simulink library "carnotUIBK"  (R2024b)
settings: Solver=VariableStepAuto  StartTime=0.0  StopTime=10.0  RelTol=1e-3  EnableMultiTasking=on
values from neighbouring files (symbols this model uses):
  area = area + room(kk).area    [THERMALZONE.m]
  boundary = BOUNDARY()    [BUILDING.m]
  building = obj    [BUILDING.m]
  C = zeros(1,length(d)+1)    [CONSTRUCTION.m]
  cp = str2num(value)    [CONSTRUCTION.m]
  pos = find(d_layer>0)    [CONSTRUCTION.m]
  rho = str2num(value)    [CONSTRUCTION.m]
  type = 1    [CONSTRUCTION.m]
  zone = obj.zone(ind)    [THERMALZONE.m]
undefined symbols (not defined in the file or in its folder): A, amb_factor, B, const, control, Dd, get_building, height, p, Qdot_C, Qdot_H, Qdot_I_electricity, Qdot_I_light, Qdot_I_person, Qdot_S, Qdot_T_ground, Qdot_T_neighbour, Qdot_T_opaque, Qdot_T_window, Qdot_V_infiltration, Qdot_V_mech, Qdot_V_window, r_frame, solar_ratio, solar_ratio1, solar_ratio2, Tc, Tr, Ts, Uvalue, view_factor, wall, wallsurface, window, window_height, window_heigth, window_width, windowsurface, x_CO2, x_H2O, x_VOC, z
libraries: carnot x105, $bdroot x22, simulink x18, simulink_extras x14
(part 13 of 13)

== system carnotUIBK/wall_zone/hygrothermal model/alpha_e/alpha_e_INTERNAL/alpha_i/alpha_i_down ==
  note: (W/m^2)
  note: Convective and radiative heat transfer at the INDOOR SURFACE of a VERTICAL OUTER WALL
  note: CONVENTION:
      | Qdot > 0 and qdots < 0, if Ts > T (heat flows from wall surface to room node),
      | Qdot < 0 and qdots > 0, if Ts < T (heat flows from room node to wall surface).
  note: s: surface
      | c: convective
      | r: radiative
  note: dynamic, convective heat transfer coefficients according to: Glück B.: Wärmeübergangskoeffizienten an thermisch aktiven Bauteiloberflächen
      | und der Übergang zu Basiskennlinien für die Wärmestromdichte; gi Gesundheits-Ingenieur; 128. Jahrgang 2007, Heft 1, Seiten 1-10
  Ts : Inport
  AIB : Inport  Port=2
  Qdot sol : Inport  Port=3
  phis : Inport  Port=4
  1/wallsurface : Gain  Gain=1/wallsurface  SaturateOnIntegerOverflow=on  OutDataTypeStr=Inherit: Same as input  ParamDataTypeStr=Inherit: Same as input
  Add : Sum  Commented=on  Inputs=+-
  Bus Selector : BusSelector  OutputSignals=Tc,Tr,p,x_H2O
  Fcn1 : Fcn  Expr=(273.15+u(1))^4-(273.15+u(2))^4
  Gain2 : Gain  Commented=on  Gain=0.01
  Ground1 : Ground
  Ground2 : Ground
  Ground3 : Ground
  Mux : Mux  Inputs=2
  Mux1 : Mux  Inputs=[2 2 1 2 12]
  Mux2 : Mux  Inputs=2
  Mux3 : Mux  Inputs=2
  Product : Product  InputSameDT=on  RndMeth=Zero  SaturateOnIntegerOverflow=on  OutDataTypeStr=Inherit: Same as first input
  Product1 : Product  InputSameDT=on  RndMeth=Zero  SaturateOnIntegerOverflow=on  OutDataTypeStr=Inherit: Same as first input
  Product2 : Product  Commented=on  RndMeth=Zero
  Product3 : Product  Commented=on  RndMeth=Zero
  Sum : Sum  Inputs=+-  InputSameDT=on  SaturateOnIntegerOverflow=on  OutDataTypeStr=Inherit: Same as first input
  Sum2 : Sum  Inputs=+--  InputSameDT=on  SaturateOnIntegerOverflow=on  OutDataTypeStr=Inherit: Same as first input
  Switch : Switch  Commented=on  Criteria=u2 > Threshold  SaturateOnIntegerOverflow=off  InputSameDT=off
  Switch1 : Switch  SaturateOnIntegerOverflow=off  InputSameDT=off
  emission_in : Gain  Gain=emission_in  SaturateOnIntegerOverflow=on  OutDataTypeStr=Inherit: Same as input  ParamDataTypeStr=Inherit: Same as input
  heat flux downwards : Fcn  Expr=0.54*(abs(u(1)-u(2))^0.31)
  heat flux upwards : Fcn  Expr=2*(abs(u(1)-u(2))^0.31)
  lewis : Gain  Commented=on  Gain=0.000000007  SaturateOnIntegerOverflow=on  OutDataTypeStr=Inherit: Same as input  ParamDataTypeStr=Inherit: Same as input
  nomassflow : Constant  Value=0
  ps_l : Fcn  Commented=on  Expr=610.0*exp(17.08*(u)/(234.2+(u)))
  ps_s_l : Fcn  Commented=on  Expr=610.0*exp(17.08*(u)/(234.2+(u)))
  sigma : Constant  Value=5.67e-8
  view_factor : Gain  Gain=view_factor  SaturateOnIntegerOverflow=on  OutDataTypeStr=Inherit: Same as input  ParamDataTypeStr=Inherit: Same as input
  wallsurface : Gain  Gain=wallsurface  SaturateOnIntegerOverflow=on  OutDataTypeStr=Inherit: Same as input  ParamDataTypeStr=Inherit: Same as input
  wallsurface1 : Gain  Commented=on  Gain=wallsurface  SaturateOnIntegerOverflow=on  OutDataTypeStr=Inherit: Same as input  ParamDataTypeStr=Inherit: Same as input
  x2RelHum_UIBK : carnot/Basic/Material_Properties/x2RelHum  Commented=on
      settings: SourceProductName=Carnot
  qdots : Outport  InitialOutput=0  VectorParamsAs1DForOutWhenUnconnected=off
  "[S]" : Outport  Port=2  InitialOutput=0  VectorParamsAs1DForOutWhenUnconnected=off
  alpha_c : Outport  Port=3  InitialOutput=0  VectorParamsAs1DForOutWhenUnconnected=off
  phi_i_1/100 : Outport  Port=4  InitialOutput=0  VectorParamsAs1DForOutWhenUnconnected=off
  wires:
  nomassflow/1 -> Mux1/3, Switch/3
  wallsurface1/1 -> Switch/1
  view_factor/1 -> Product/1
  phis/1 -> Product3/1, Switch/2
  Add/1 -> lewis/1
  Product2/1 -> Add/2
  Product3/1 -> Add/1
  ps_s_l/1 -> Product3/2
  ps_l/1 -> Product2/2
  Ground3/1 -> Mux1/2
  Ground1/1 -> Mux1/4
  Ground2/1 -> Mux1/5
  lewis/1 -> wallsurface1/1
  Gain2/1 -> Product2/1, phi_i_1/100/1
  Bus Selector/4 -> x2RelHum_UIBK/3  "<x_H2O>"
  Bus Selector/3 -> x2RelHum_UIBK/2  "<p>"
  x2RelHum_UIBK/1 -> Gain2/1
  Fcn1/1 -> Product/2
  Mux3/1 -> Fcn1/1
  sigma/1 -> emission_in/1
  Mux1/1 -> "[S]"/1
  Sum2/1 -> qdots/1
  AIB/1 -> Bus Selector/1
  Bus Selector/1 -> Sum/2, Mux2/2, x2RelHum_UIBK/1, ps_l/1  "<Tc>"
  emission_in/1 -> view_factor/1
  Product/1 -> Sum2/3, Mux/2  "qdotr"
  Mux/1 -> wallsurface/1
  Ts/1 -> Sum/1, ps_s_l/1, Mux3/1, Mux2/1  "Ts"
  Bus Selector/2 -> Mux3/2  "<Tr>"
  Mux2/1 -> heat flux downwards/1, heat flux upwards/1
  Product1/1 -> Mux/1, Sum2/2  "qdotc"
  Switch1/1 -> Product1/2, alpha_c/1  "hc"
  wallsurface/1 -> Mux1/1  "[Qdotc, Qdotr]"
  Qdot sol/1 -> 1/wallsurface/1
  1/wallsurface/1 -> Sum2/1
  Sum/1 -> Switch1/2, Product1/1  "dTc"
  heat flux upwards/1 -> Switch1/1
  heat flux downwards/1 -> Switch1/3

== system carnotUIBK/wall_zone/hygrothermal model/alpha_e/alpha_e_INTERNAL/alpha_i/alpha_i_horizontal ==
  note: (W/m^2)
  note: Convective and radiative heat transfer at the INDOOR SURFACE of a VERTICAL OUTER WALL
  note: CONVENTION:
      | Qdot > 0 and qdots < 0, if Ts > T (heat flows from wall surface to room node),
      | Qdot < 0 and qdots > 0, if Ts < T (heat flows from room node to wall surface).
  note: s: surface
      | c: convective
      | r: radiative
  note: dynamic, convective heat transfer coefficients according to: Glück B.: Wärmeübergangskoeffizienten an thermisch aktiven Bauteiloberflächen
      | und der Übergang zu Basiskennlinien für die Wärmestromdichte; gi Gesundheits-Ingenieur; 128. Jahrgang 2007, Heft 1, Seiten 1-10
  Ts : Inport
  AIB : Inport  Port=2
  Qdot sol : Inport  Port=3
  phis : Inport  Port=4
  1/wallsurface : Gain  Gain=1/wallsurface  SaturateOnIntegerOverflow=on  OutDataTypeStr=Inherit: Same as input  ParamDataTypeStr=Inherit: Same as input
  Add : Sum  Commented=on  Inputs=+-
  Bus Selector : BusSelector  OutputSignals=Tc,Tr,p,x_H2O
  Fcn : Fcn  Expr=1.6*(abs(u(1)-u(2)))^0.3
  Fcn1 : Fcn  Expr=(273.15+u(1))^4-(273.15+u(2))^4
  Gain2 : Gain  Commented=on  Gain=0.01
  Ground1 : Ground
  Ground2 : Ground
  Ground3 : Ground
  Mux : Mux  Inputs=2
  Mux1 : Mux  Inputs=[2 2 1 2 12]
  Mux2 : Mux  Inputs=2
  Mux3 : Mux  Inputs=2
  Product : Product  InputSameDT=on  RndMeth=Zero  SaturateOnIntegerOverflow=on  OutDataTypeStr=Inherit: Same as first input
  Product1 : Product  InputSameDT=on  RndMeth=Zero  SaturateOnIntegerOverflow=on  OutDataTypeStr=Inherit: Same as first input
  Product2 : Product  Commented=on  RndMeth=Zero
  Product3 : Product  Commented=on  RndMeth=Zero
  Sum : Sum  Inputs=+-  InputSameDT=on  SaturateOnIntegerOverflow=on  OutDataTypeStr=Inherit: Same as first input
  Sum2 : Sum  Inputs=+--  InputSameDT=on  SaturateOnIntegerOverflow=on  OutDataTypeStr=Inherit: Same as first input
  Switch : Switch  Commented=on  Criteria=u2 > Threshold  SaturateOnIntegerOverflow=off  InputSameDT=off
  emission_in : Gain  Gain=emission_in  SaturateOnIntegerOverflow=on  OutDataTypeStr=Inherit: Same as input  ParamDataTypeStr=Inherit: Same as input
  lewis : Gain  Commented=on  Gain=0.000000007  SaturateOnIntegerOverflow=on  OutDataTypeStr=Inherit: Same as input  ParamDataTypeStr=Inherit: Same as input
  nomassflow : Constant  Value=0
  ps_l : Fcn  Commented=on  Expr=610.0*exp(17.08*(u)/(234.2+(u)))
  ps_s_l : Fcn  Commented=on  Expr=610.0*exp(17.08*(u)/(234.2+(u)))
  sigma : Constant  Value=5.67e-8
  view_factor : Gain  Gain=view_factor  SaturateOnIntegerOverflow=on  OutDataTypeStr=Inherit: Same as input  ParamDataTypeStr=Inherit: Same as input
  wallsurface : Gain  Gain=wallsurface  SaturateOnIntegerOverflow=on  OutDataTypeStr=Inherit: Same as input  ParamDataTypeStr=Inherit: Same as input
  wallsurface1 : Gain  Commented=on  Gain=wallsurface  SaturateOnIntegerOverflow=on  OutDataTypeStr=Inherit: Same as input  ParamDataTypeStr=Inherit: Same as input
  x2RelHum_UIBK : carnot/Basic/Material_Properties/x2RelHum  Commented=on
      settings: SourceProductName=Carnot
  qdots : Outport  InitialOutput=0  VectorParamsAs1DForOutWhenUnconnected=off
  "[S]" : Outport  Port=2  InitialOutput=0  VectorParamsAs1DForOutWhenUnconnected=off
  alpha_c : Outport  Port=3  InitialOutput=0  VectorParamsAs1DForOutWhenUnconnected=off
  phi_i_1/100 : Outport  Port=4  InitialOutput=0  VectorParamsAs1DForOutWhenUnconnected=off
  wires:
  nomassflow/1 -> Mux1/3, Switch/3
  wallsurface1/1 -> Switch/1
  view_factor/1 -> Product/1
  phis/1 -> Product3/1, Switch/2
  Add/1 -> lewis/1
  Product2/1 -> Add/2
  Product3/1 -> Add/1
  ps_s_l/1 -> Product3/2
  ps_l/1 -> Product2/2
  Ground3/1 -> Mux1/2
  Ground1/1 -> Mux1/4
  Ground2/1 -> Mux1/5
  lewis/1 -> wallsurface1/1
  Gain2/1 -> Product2/1, phi_i_1/100/1
  Bus Selector/4 -> x2RelHum_UIBK/3  "<x_H2O>"
  Bus Selector/3 -> x2RelHum_UIBK/2  "<p>"
  x2RelHum_UIBK/1 -> Gain2/1
  Fcn1/1 -> Product/2
  Mux3/1 -> Fcn1/1
  sigma/1 -> emission_in/1
  Mux1/1 -> "[S]"/1
  Sum2/1 -> qdots/1
  AIB/1 -> Bus Selector/1
  Bus Selector/1 -> Sum/2, Mux2/2, x2RelHum_UIBK/1, ps_l/1  "<Tc>"
  emission_in/1 -> view_factor/1
  Product/1 -> Sum2/3, Mux/2  "qdotr"
  Mux/1 -> wallsurface/1
  Ts/1 -> Sum/1, ps_s_l/1, Mux3/1, Mux2/1  "Ts"
  Sum/1 -> Product1/1  "dTc"
  Bus Selector/2 -> Mux3/2  "<Tr>"
  Mux2/1 -> Fcn/1
  Product1/1 -> Mux/1, Sum2/2  "qdotc"
  Fcn/1 -> alpha_c/1, Product1/2  "hc"
  wallsurface/1 -> Mux1/1  "[Qdotc, Qdotr]"
  Qdot sol/1 -> 1/wallsurface/1
  1/wallsurface/1 -> Sum2/1

== system carnotUIBK/wall_zone/hygrothermal model/alpha_e/alpha_e_INTERNAL/alpha_i/alpha_i_up ==
  note: (W/m^2)
  note: Convective and radiative heat transfer at the INDOOR SURFACE of a VERTICAL OUTER WALL
  note: CONVENTION:
      | Qdot > 0 and qdots < 0, if Ts > T (heat flows from wall surface to room node),
      | Qdot < 0 and qdots > 0, if Ts < T (heat flows from room node to wall surface).
  note: s: surface
      | c: convective
      | r: radiative
  note: dynamic, convective heat transfer coefficients according to: Glück B.: Wärmeübergangskoeffizienten an thermisch aktiven Bauteiloberflächen
      | und der Übergang zu Basiskennlinien für die Wärmestromdichte; gi Gesundheits-Ingenieur; 128. Jahrgang 2007, Heft 1, Seiten 1-10
  Ts : Inport
  AIB : Inport  Port=2
  Qdot sol : Inport  Port=3
  phis : Inport  Port=4
  1/wallsurface : Gain  Gain=1/wallsurface  SaturateOnIntegerOverflow=on  OutDataTypeStr=Inherit: Same as input  ParamDataTypeStr=Inherit: Same as input
  Add : Sum  Commented=on  Inputs=+-
  Bus Selector : BusSelector  OutputSignals=Tc,Tr,p,x_H2O
  Fcn1 : Fcn  Expr=(273.15+u(1))^4-(273.15+u(2))^4
  Gain2 : Gain  Commented=on  Gain=0.01
  Ground1 : Ground
  Ground2 : Ground
  Ground3 : Ground
  Mux : Mux  Inputs=2
  Mux1 : Mux  Inputs=[2 2 1 2 12]
  Mux2 : Mux  Inputs=2
  Mux3 : Mux  Inputs=2
  Product : Product  InputSameDT=on  RndMeth=Zero  SaturateOnIntegerOverflow=on  OutDataTypeStr=Inherit: Same as first input
  Product1 : Product  InputSameDT=on  RndMeth=Zero  SaturateOnIntegerOverflow=on  OutDataTypeStr=Inherit: Same as first input
  Product2 : Product  Commented=on  RndMeth=Zero
  Product3 : Product  Commented=on  RndMeth=Zero
  Sum : Sum  Inputs=+-  InputSameDT=on  SaturateOnIntegerOverflow=on  OutDataTypeStr=Inherit: Same as first input
  Sum2 : Sum  Inputs=+--  InputSameDT=on  SaturateOnIntegerOverflow=on  OutDataTypeStr=Inherit: Same as first input
  Switch : Switch  Commented=on  Criteria=u2 > Threshold  SaturateOnIntegerOverflow=off  InputSameDT=off
  Switch1 : Switch  SaturateOnIntegerOverflow=off  InputSameDT=off
  emission_in : Gain  Gain=emission_in  SaturateOnIntegerOverflow=on  OutDataTypeStr=Inherit: Same as input  ParamDataTypeStr=Inherit: Same as input
  heat flux downwards : Fcn  Expr=0.54*(abs(u(1)-u(2))^0.31)
  heat flux upwards : Fcn  Expr=2*(abs(u(1)-u(2))^0.31)
  lewis : Gain  Commented=on  Gain=0.000000007  SaturateOnIntegerOverflow=on  OutDataTypeStr=Inherit: Same as input  ParamDataTypeStr=Inherit: Same as input
  nomassflow : Constant  Value=0
  ps_l : Fcn  Commented=on  Expr=610.0*exp(17.08*(u)/(234.2+(u)))
  ps_s_l : Fcn  Commented=on  Expr=610.0*exp(17.08*(u)/(234.2+(u)))
  sigma : Constant  Value=5.67e-8
  view_factor : Gain  Gain=view_factor  SaturateOnIntegerOverflow=on  OutDataTypeStr=Inherit: Same as input  ParamDataTypeStr=Inherit: Same as input
  wallsurface : Gain  Gain=wallsurface  SaturateOnIntegerOverflow=on  OutDataTypeStr=Inherit: Same as input  ParamDataTypeStr=Inherit: Same as input
  wallsurface1 : Gain  Commented=on  Gain=wallsurface  SaturateOnIntegerOverflow=on  OutDataTypeStr=Inherit: Same as input  ParamDataTypeStr=Inherit: Same as input
  x2RelHum_UIBK : carnot/Basic/Material_Properties/x2RelHum  Commented=on
      settings: SourceProductName=Carnot
  qdots : Outport  InitialOutput=0  VectorParamsAs1DForOutWhenUnconnected=off
  "[S]" : Outport  Port=2  InitialOutput=0  VectorParamsAs1DForOutWhenUnconnected=off
  alpha_c : Outport  Port=3  InitialOutput=0  VectorParamsAs1DForOutWhenUnconnected=off
  phi_i_1/100 : Outport  Port=4  InitialOutput=0  VectorParamsAs1DForOutWhenUnconnected=off
  wires:
  nomassflow/1 -> Mux1/3, Switch/3
  wallsurface1/1 -> Switch/1
  view_factor/1 -> Product/1
  phis/1 -> Product3/1, Switch/2
  Add/1 -> lewis/1
  Product2/1 -> Add/2
  Product3/1 -> Add/1
  ps_s_l/1 -> Product3/2
  ps_l/1 -> Product2/2
  Ground3/1 -> Mux1/2
  Ground1/1 -> Mux1/4
  Ground2/1 -> Mux1/5
  lewis/1 -> wallsurface1/1
  Gain2/1 -> Product2/1, phi_i_1/100/1
  Bus Selector/4 -> x2RelHum_UIBK/3  "<x_H2O>"
  Bus Selector/3 -> x2RelHum_UIBK/2  "<p>"
  x2RelHum_UIBK/1 -> Gain2/1
  Fcn1/1 -> Product/2
  Mux3/1 -> Fcn1/1
  sigma/1 -> emission_in/1
  Mux1/1 -> "[S]"/1
  Sum2/1 -> qdots/1
  AIB/1 -> Bus Selector/1
  Bus Selector/1 -> Sum/2, Mux2/2, x2RelHum_UIBK/1, ps_l/1  "<Tc>"
  emission_in/1 -> view_factor/1
  Product/1 -> Sum2/3, Mux/2  "qdotr"
  Mux/1 -> wallsurface/1
  Ts/1 -> Sum/1, ps_s_l/1, Mux3/1, Mux2/1  "Ts"
  Bus Selector/2 -> Mux3/2  "<Tr>"
  Mux2/1 -> heat flux downwards/1, heat flux upwards/1
  Product1/1 -> Mux/1, Sum2/2  "qdotc"
  Switch1/1 -> Product1/2, alpha_c/1  "hc"
  wallsurface/1 -> Mux1/1  "[Qdotc, Qdotr]"
  Qdot sol/1 -> 1/wallsurface/1
  1/wallsurface/1 -> Sum2/1
  Sum/1 -> Switch1/2, Product1/1  "dTc"
  heat flux upwards/1 -> Switch1/1
  heat flux downwards/1 -> Switch1/3

== system carnotUIBK/wall_zone/hygrothermal model/alpha_e/alpha_e_NEIGHBOUR/alpha_i/alpha_i_down ==
  note: (W/m^2)
  note: Convective and radiative heat transfer at the INDOOR SURFACE of a VERTICAL OUTER WALL
  note: CONVENTION:
      | Qdot > 0 and qdots < 0, if Ts > T (heat flows from wall surface to room node),
      | Qdot < 0 and qdots > 0, if Ts < T (heat flows from room node to wall surface).
  note: s: surface
      | c: convective
      | r: radiative
  note: dynamic, convective heat transfer coefficients according to: Glück B.: Wärmeübergangskoeffizienten an thermisch aktiven Bauteiloberflächen
      | und der Übergang zu Basiskennlinien für die Wärmestromdichte; gi Gesundheits-Ingenieur; 128. Jahrgang 2007, Heft 1, Seiten 1-10
  Ts : Inport
  AIB : Inport  Port=2
  Qdot sol : Inport  Port=3
  phis : Inport  Port=4
  1/wallsurface : Gain  Gain=1/wallsurface  SaturateOnIntegerOverflow=on  OutDataTypeStr=Inherit: Same as input  ParamDataTypeStr=Inherit: Same as input
  Add : Sum  Commented=on  Inputs=+-
  Bus Selector : BusSelector  OutputSignals=Tc,Tr,p,x_H2O
  Fcn1 : Fcn  Expr=(273.15+u(1))^4-(273.15+u(2))^4
  Gain2 : Gain  Commented=on  Gain=0.01
  Ground1 : Ground
  Ground2 : Ground
  Ground3 : Ground
  Mux : Mux  Inputs=2
  Mux1 : Mux  Inputs=[2 2 1 2 12]
  Mux2 : Mux  Inputs=2
  Mux3 : Mux  Inputs=2
  Product : Product  InputSameDT=on  RndMeth=Zero  SaturateOnIntegerOverflow=on  OutDataTypeStr=Inherit: Same as first input
  Product1 : Product  InputSameDT=on  RndMeth=Zero  SaturateOnIntegerOverflow=on  OutDataTypeStr=Inherit: Same as first input
  Product2 : Product  Commented=on  RndMeth=Zero
  Product3 : Product  Commented=on  RndMeth=Zero
  Sum : Sum  Inputs=+-  InputSameDT=on  SaturateOnIntegerOverflow=on  OutDataTypeStr=Inherit: Same as first input
  Sum2 : Sum  Inputs=+--  InputSameDT=on  SaturateOnIntegerOverflow=on  OutDataTypeStr=Inherit: Same as first input
  Switch : Switch  Commented=on  Criteria=u2 > Threshold  SaturateOnIntegerOverflow=off  InputSameDT=off
  Switch1 : Switch  SaturateOnIntegerOverflow=off  InputSameDT=off
  emission_in : Gain  Gain=emission_in  SaturateOnIntegerOverflow=on  OutDataTypeStr=Inherit: Same as input  ParamDataTypeStr=Inherit: Same as input
  heat flux downwards : Fcn  Expr=0.54*(abs(u(1)-u(2))^0.31)
  heat flux upwards : Fcn  Expr=2*(abs(u(1)-u(2))^0.31)
  lewis : Gain  Commented=on  Gain=0.000000007  SaturateOnIntegerOverflow=on  OutDataTypeStr=Inherit: Same as input  ParamDataTypeStr=Inherit: Same as input
  nomassflow : Constant  Value=0
  ps_l : Fcn  Commented=on  Expr=610.0*exp(17.08*(u)/(234.2+(u)))
  ps_s_l : Fcn  Commented=on  Expr=610.0*exp(17.08*(u)/(234.2+(u)))
  sigma : Constant  Value=5.67e-8
  view_factor : Gain  Gain=view_factor  SaturateOnIntegerOverflow=on  OutDataTypeStr=Inherit: Same as input  ParamDataTypeStr=Inherit: Same as input
  wallsurface : Gain  Gain=wallsurface  SaturateOnIntegerOverflow=on  OutDataTypeStr=Inherit: Same as input  ParamDataTypeStr=Inherit: Same as input
  wallsurface1 : Gain  Commented=on  Gain=wallsurface  SaturateOnIntegerOverflow=on  OutDataTypeStr=Inherit: Same as input  ParamDataTypeStr=Inherit: Same as input
  x2RelHum_UIBK : carnot/Basic/Material_Properties/x2RelHum  Commented=on
      settings: SourceProductName=Carnot
  qdots : Outport  InitialOutput=0  VectorParamsAs1DForOutWhenUnconnected=off
  "[S]" : Outport  Port=2  InitialOutput=0  VectorParamsAs1DForOutWhenUnconnected=off
  alpha_c : Outport  Port=3  InitialOutput=0  VectorParamsAs1DForOutWhenUnconnected=off
  phi_i_1/100 : Outport  Port=4  InitialOutput=0  VectorParamsAs1DForOutWhenUnconnected=off
  wires:
  nomassflow/1 -> Mux1/3, Switch/3
  wallsurface1/1 -> Switch/1
  view_factor/1 -> Product/1
  phis/1 -> Product3/1, Switch/2
  Add/1 -> lewis/1
  Product2/1 -> Add/2
  Product3/1 -> Add/1
  ps_s_l/1 -> Product3/2
  ps_l/1 -> Product2/2
  Ground3/1 -> Mux1/2
  Ground1/1 -> Mux1/4
  Ground2/1 -> Mux1/5
  lewis/1 -> wallsurface1/1
  Gain2/1 -> Product2/1, phi_i_1/100/1
  Bus Selector/4 -> x2RelHum_UIBK/3  "<x_H2O>"
  Bus Selector/3 -> x2RelHum_UIBK/2  "<p>"
  x2RelHum_UIBK/1 -> Gain2/1
  Fcn1/1 -> Product/2
  Mux3/1 -> Fcn1/1
  sigma/1 -> emission_in/1
  Mux1/1 -> "[S]"/1
  Sum2/1 -> qdots/1
  AIB/1 -> Bus Selector/1
  Bus Selector/1 -> Sum/2, Mux2/2, x2RelHum_UIBK/1, ps_l/1  "<Tc>"
  emission_in/1 -> view_factor/1
  Product/1 -> Sum2/3, Mux/2  "qdotr"
  Mux/1 -> wallsurface/1
  Ts/1 -> Sum/1, ps_s_l/1, Mux3/1, Mux2/1  "Ts"
  Bus Selector/2 -> Mux3/2  "<Tr>"
  Mux2/1 -> heat flux downwards/1, heat flux upwards/1
  Product1/1 -> Mux/1, Sum2/2  "qdotc"
  Switch1/1 -> Product1/2, alpha_c/1  "hc"
  wallsurface/1 -> Mux1/1  "[Qdotc, Qdotr]"
  Qdot sol/1 -> 1/wallsurface/1
  1/wallsurface/1 -> Sum2/1
  Sum/1 -> Switch1/2, Product1/1  "dTc"
  heat flux upwards/1 -> Switch1/1
  heat flux downwards/1 -> Switch1/3

== system carnotUIBK/wall_zone/hygrothermal model/alpha_e/alpha_e_NEIGHBOUR/alpha_i/alpha_i_horizontal ==
  note: (W/m^2)
  note: Convective and radiative heat transfer at the INDOOR SURFACE of a VERTICAL OUTER WALL
  note: CONVENTION:
      | Qdot > 0 and qdots < 0, if Ts > T (heat flows from wall surface to room node),
      | Qdot < 0 and qdots > 0, if Ts < T (heat flows from room node to wall surface).
  note: s: surface
      | c: convective
      | r: radiative
  note: dynamic, convective heat transfer coefficients according to: Glück B.: Wärmeübergangskoeffizienten an thermisch aktiven Bauteiloberflächen
      | und der Übergang zu Basiskennlinien für die Wärmestromdichte; gi Gesundheits-Ingenieur; 128. Jahrgang 2007, Heft 1, Seiten 1-10
  Ts : Inport
  AIB : Inport  Port=2
  Qdot sol : Inport  Port=3
  phis : Inport  Port=4
  1/wallsurface : Gain  Gain=1/wallsurface  SaturateOnIntegerOverflow=on  OutDataTypeStr=Inherit: Same as input  ParamDataTypeStr=Inherit: Same as input
  Add : Sum  Commented=on  Inputs=+-
  Bus Selector : BusSelector  OutputSignals=Tc,Tr,p,x_H2O
  Fcn : Fcn  Expr=1.6*(abs(u(1)-u(2)))^0.3
  Fcn1 : Fcn  Expr=(273.15+u(1))^4-(273.15+u(2))^4
  Gain2 : Gain  Commented=on  Gain=0.01
  Ground1 : Ground
  Ground2 : Ground
  Ground3 : Ground
  Mux : Mux  Inputs=2
  Mux1 : Mux  Inputs=[2 2 1 2 12]
  Mux2 : Mux  Inputs=2
  Mux3 : Mux  Inputs=2
  Product : Product  InputSameDT=on  RndMeth=Zero  SaturateOnIntegerOverflow=on  OutDataTypeStr=Inherit: Same as first input
  Product1 : Product  InputSameDT=on  RndMeth=Zero  SaturateOnIntegerOverflow=on  OutDataTypeStr=Inherit: Same as first input
  Product2 : Product  Commented=on  RndMeth=Zero
  Product3 : Product  Commented=on  RndMeth=Zero
  Sum : Sum  Inputs=+-  InputSameDT=on  SaturateOnIntegerOverflow=on  OutDataTypeStr=Inherit: Same as first input
  Sum2 : Sum  Inputs=+--  InputSameDT=on  SaturateOnIntegerOverflow=on  OutDataTypeStr=Inherit: Same as first input
  Switch : Switch  Commented=on  Criteria=u2 > Threshold  SaturateOnIntegerOverflow=off  InputSameDT=off
  emission_in : Gain  Gain=emission_in  SaturateOnIntegerOverflow=on  OutDataTypeStr=Inherit: Same as input  ParamDataTypeStr=Inherit: Same as input
  lewis : Gain  Commented=on  Gain=0.000000007  SaturateOnIntegerOverflow=on  OutDataTypeStr=Inherit: Same as input  ParamDataTypeStr=Inherit: Same as input
  nomassflow : Constant  Value=0
  ps_l : Fcn  Commented=on  Expr=610.0*exp(17.08*(u)/(234.2+(u)))
  ps_s_l : Fcn  Commented=on  Expr=610.0*exp(17.08*(u)/(234.2+(u)))
  sigma : Constant  Value=5.67e-8
  view_factor : Gain  Gain=view_factor  SaturateOnIntegerOverflow=on  OutDataTypeStr=Inherit: Same as input  ParamDataTypeStr=Inherit: Same as input
  wallsurface : Gain  Gain=wallsurface  SaturateOnIntegerOverflow=on  OutDataTypeStr=Inherit: Same as input  ParamDataTypeStr=Inherit: Same as input
  wallsurface1 : Gain  Commented=on  Gain=wallsurface  SaturateOnIntegerOverflow=on  OutDataTypeStr=Inherit: Same as input  ParamDataTypeStr=Inherit: Same as input
  x2RelHum_UIBK : carnot/Basic/Material_Properties/x2RelHum  Commented=on
      settings: SourceProductName=Carnot
  qdots : Outport  InitialOutput=0  VectorParamsAs1DForOutWhenUnconnected=off
  "[S]" : Outport  Port=2  InitialOutput=0  VectorParamsAs1DForOutWhenUnconnected=off
  alpha_c : Outport  Port=3  InitialOutput=0  VectorParamsAs1DForOutWhenUnconnected=off
  phi_i_1/100 : Outport  Port=4  InitialOutput=0  VectorParamsAs1DForOutWhenUnconnected=off
  wires:
  nomassflow/1 -> Mux1/3, Switch/3
  wallsurface1/1 -> Switch/1
  view_factor/1 -> Product/1
  phis/1 -> Product3/1, Switch/2
  Add/1 -> lewis/1
  Product2/1 -> Add/2
  Product3/1 -> Add/1
  ps_s_l/1 -> Product3/2
  ps_l/1 -> Product2/2
  Ground3/1 -> Mux1/2
  Ground1/1 -> Mux1/4
  Ground2/1 -> Mux1/5
  lewis/1 -> wallsurface1/1
  Gain2/1 -> Product2/1, phi_i_1/100/1
  Bus Selector/4 -> x2RelHum_UIBK/3  "<x_H2O>"
  Bus Selector/3 -> x2RelHum_UIBK/2  "<p>"
  x2RelHum_UIBK/1 -> Gain2/1
  Fcn1/1 -> Product/2
  Mux3/1 -> Fcn1/1
  sigma/1 -> emission_in/1
  Mux1/1 -> "[S]"/1
  Sum2/1 -> qdots/1
  AIB/1 -> Bus Selector/1
  Bus Selector/1 -> Sum/2, Mux2/2, x2RelHum_UIBK/1, ps_l/1  "<Tc>"
  emission_in/1 -> view_factor/1
  Product/1 -> Sum2/3, Mux/2  "qdotr"
  Mux/1 -> wallsurface/1
  Ts/1 -> Sum/1, ps_s_l/1, Mux3/1, Mux2/1  "Ts"
  Sum/1 -> Product1/1  "dTc"
  Bus Selector/2 -> Mux3/2  "<Tr>"
  Mux2/1 -> Fcn/1
  Product1/1 -> Mux/1, Sum2/2  "qdotc"
  Fcn/1 -> alpha_c/1, Product1/2  "hc"
  wallsurface/1 -> Mux1/1  "[Qdotc, Qdotr]"
  Qdot sol/1 -> 1/wallsurface/1
  1/wallsurface/1 -> Sum2/1

== system carnotUIBK/wall_zone/hygrothermal model/alpha_e/alpha_e_NEIGHBOUR/alpha_i/alpha_i_up ==
  note: (W/m^2)
  note: Convective and radiative heat transfer at the INDOOR SURFACE of a VERTICAL OUTER WALL
  note: CONVENTION:
      | Qdot > 0 and qdots < 0, if Ts > T (heat flows from wall surface to room node),
      | Qdot < 0 and qdots > 0, if Ts < T (heat flows from room node to wall surface).
  note: s: surface
      | c: convective
      | r: radiative
  note: dynamic, convective heat transfer coefficients according to: Glück B.: Wärmeübergangskoeffizienten an thermisch aktiven Bauteiloberflächen
      | und der Übergang zu Basiskennlinien für die Wärmestromdichte; gi Gesundheits-Ingenieur; 128. Jahrgang 2007, Heft 1, Seiten 1-10
  Ts : Inport
  AIB : Inport  Port=2
  Qdot sol : Inport  Port=3
  phis : Inport  Port=4
  1/wallsurface : Gain  Gain=1/wallsurface  SaturateOnIntegerOverflow=on  OutDataTypeStr=Inherit: Same as input  ParamDataTypeStr=Inherit: Same as input
  Add : Sum  Commented=on  Inputs=+-
  Bus Selector : BusSelector  OutputSignals=Tc,Tr,p,x_H2O
  Fcn1 : Fcn  Expr=(273.15+u(1))^4-(273.15+u(2))^4
  Gain2 : Gain  Commented=on  Gain=0.01
  Ground1 : Ground
  Ground2 : Ground
  Ground3 : Ground
  Mux : Mux  Inputs=2
  Mux1 : Mux  Inputs=[2 2 1 2 12]
  Mux2 : Mux  Inputs=2
  Mux3 : Mux  Inputs=2
  Product : Product  InputSameDT=on  RndMeth=Zero  SaturateOnIntegerOverflow=on  OutDataTypeStr=Inherit: Same as first input
  Product1 : Product  InputSameDT=on  RndMeth=Zero  SaturateOnIntegerOverflow=on  OutDataTypeStr=Inherit: Same as first input
  Product2 : Product  Commented=on  RndMeth=Zero
  Product3 : Product  Commented=on  RndMeth=Zero
  Sum : Sum  Inputs=+-  InputSameDT=on  SaturateOnIntegerOverflow=on  OutDataTypeStr=Inherit: Same as first input
  Sum2 : Sum  Inputs=+--  InputSameDT=on  SaturateOnIntegerOverflow=on  OutDataTypeStr=Inherit: Same as first input
  Switch : Switch  Commented=on  Criteria=u2 > Threshold  SaturateOnIntegerOverflow=off  InputSameDT=off
  Switch1 : Switch  SaturateOnIntegerOverflow=off  InputSameDT=off
  emission_in : Gain  Gain=emission_in  SaturateOnIntegerOverflow=on  OutDataTypeStr=Inherit: Same as input  ParamDataTypeStr=Inherit: Same as input
  heat flux downwards : Fcn  Expr=0.54*(abs(u(1)-u(2))^0.31)
  heat flux upwards : Fcn  Expr=2*(abs(u(1)-u(2))^0.31)
  lewis : Gain  Commented=on  Gain=0.000000007  SaturateOnIntegerOverflow=on  OutDataTypeStr=Inherit: Same as input  ParamDataTypeStr=Inherit: Same as input
  nomassflow : Constant  Value=0
  ps_l : Fcn  Commented=on  Expr=610.0*exp(17.08*(u)/(234.2+(u)))
  ps_s_l : Fcn  Commented=on  Expr=610.0*exp(17.08*(u)/(234.2+(u)))
  sigma : Constant  Value=5.67e-8
  view_factor : Gain  Gain=view_factor  SaturateOnIntegerOverflow=on  OutDataTypeStr=Inherit: Same as input  ParamDataTypeStr=Inherit: Same as input
  wallsurface : Gain  Gain=wallsurface  SaturateOnIntegerOverflow=on  OutDataTypeStr=Inherit: Same as input  ParamDataTypeStr=Inherit: Same as input
  wallsurface1 : Gain  Commented=on  Gain=wallsurface  SaturateOnIntegerOverflow=on  OutDataTypeStr=Inherit: Same as input  ParamDataTypeStr=Inherit: Same as input
  x2RelHum_UIBK : carnot/Basic/Material_Properties/x2RelHum  Commented=on
      settings: SourceProductName=Carnot
  qdots : Outport  InitialOutput=0  VectorParamsAs1DForOutWhenUnconnected=off
  "[S]" : Outport  Port=2  InitialOutput=0  VectorParamsAs1DForOutWhenUnconnected=off
  alpha_c : Outport  Port=3  InitialOutput=0  VectorParamsAs1DForOutWhenUnconnected=off
  phi_i_1/100 : Outport  Port=4  InitialOutput=0  VectorParamsAs1DForOutWhenUnconnected=off
  wires:
  nomassflow/1 -> Mux1/3, Switch/3
  wallsurface1/1 -> Switch/1
  view_factor/1 -> Product/1
  phis/1 -> Product3/1, Switch/2
  Add/1 -> lewis/1
  Product2/1 -> Add/2
  Product3/1 -> Add/1
  ps_s_l/1 -> Product3/2
  ps_l/1 -> Product2/2
  Ground3/1 -> Mux1/2
  Ground1/1 -> Mux1/4
  Ground2/1 -> Mux1/5
  lewis/1 -> wallsurface1/1
  Gain2/1 -> Product2/1, phi_i_1/100/1
  Bus Selector/4 -> x2RelHum_UIBK/3  "<x_H2O>"
  Bus Selector/3 -> x2RelHum_UIBK/2  "<p>"
  x2RelHum_UIBK/1 -> Gain2/1
  Fcn1/1 -> Product/2
  Mux3/1 -> Fcn1/1
  sigma/1 -> emission_in/1
  Mux1/1 -> "[S]"/1
  Sum2/1 -> qdots/1
  AIB/1 -> Bus Selector/1
  Bus Selector/1 -> Sum/2, Mux2/2, x2RelHum_UIBK/1, ps_l/1  "<Tc>"
  emission_in/1 -> view_factor/1
  Product/1 -> Sum2/3, Mux/2  "qdotr"
  Mux/1 -> wallsurface/1
  Ts/1 -> Sum/1, ps_s_l/1, Mux3/1, Mux2/1  "Ts"
  Bus Selector/2 -> Mux3/2  "<Tr>"
  Mux2/1 -> heat flux downwards/1, heat flux upwards/1
  Product1/1 -> Mux/1, Sum2/2  "qdotc"
  Switch1/1 -> Product1/2, alpha_c/1  "hc"
  wallsurface/1 -> Mux1/1  "[Qdotc, Qdotr]"
  Qdot sol/1 -> 1/wallsurface/1
  1/wallsurface/1 -> Sum2/1
  Sum/1 -> Switch1/2, Product1/1  "dTc"
  heat flux upwards/1 -> Switch1/1
  heat flux downwards/1 -> Switch1/3

== system carnotUIBK/window/window_CARNOT/alfa_window_in/transmission coefficient 1-2-3-4-layer(s)/LUT_taualfa/TAUALFA 1-2-3-4 layers, standardized to 1.0, (4 mm float glass, no dirt absorption, 97% room absorption) ==
  Rows : Inport
  Cols : Inport  Port=2
  Look-Up Table (2-D) : Lookup2D  RowIndex=x  ColumnIndex=y  Table=t
  Out1 : Outport  VectorParamsAs1DForOutWhenUnconnected=off
  wires:
  Rows/1 -> Look-Up Table (2-D)/1
  Cols/1 -> Look-Up Table (2-D)/2
  Look-Up Table (2-D)/1 -> Out1/1
